simulink model "sistemaDesacopladoEquivalenteControlCorriente"  (R2012b)
settings: Solver=ode45  StartTime=0.0  StopTime=10.0  RelTol=1e-3
values from neighbouring files (symbols this model uses):
  b_m = bm+(bl/r^2)    (= 1.5e-05)    [InicializaYconstantes.m]
  J_m = Jm+(Jl/r^2)    (= 5.65099476805e-06)    [InicializaYconstantes.m]
  lambda = 0.01546    [InicializaYconstantes.m]
  Ld = 6.6*10^-3    (= 0.0066)    [InicializaYconstantes.m]
  Lq = 5.8*10^-3    (= 0.0058)    [InicializaYconstantes.m]
  Pp = 3    [InicializaYconstantes.m]
  R1 = -p1i*Lq    (= 29)    [InicializaYconstantes.m]
  R2 = -p1i*Ld    (= 33)    [InicializaYconstantes.m]
  T_l = Tl/r    (= 0.00499521477515)    [InicializaYconstantes.m]
settings Model: Creator=usuario  LastModifiedBy=usuario

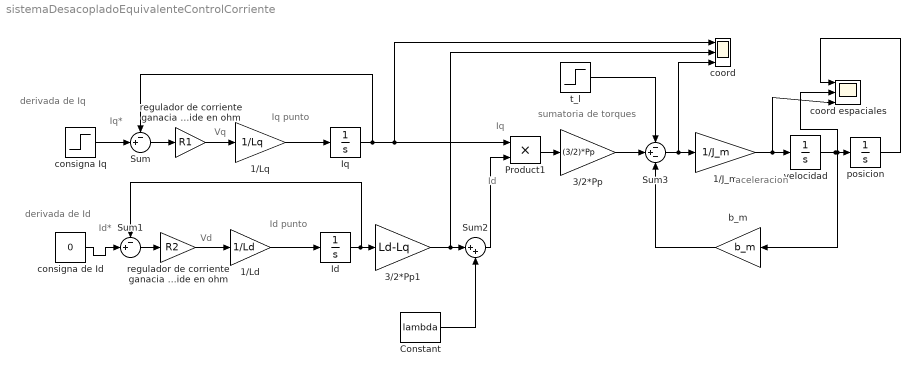
== system sistemaDesacopladoEquivalenteControlCorriente ==
  note: derivada de Id
  note: derivada de Iq
  note: Id*
  note: Iq*
  note: Vd
  note: Vq
  note: sumatoria de torques
  note: Iq
  note: aceleracion
  note: Id
  note: Iq punto
  note: Id punto
  1/J_m : Gain  Gain=1/J_m
  1/Ld : Gain  Gain=1/Ld
  1/Lq : Gain  Gain=1/Lq
  3/2*Pp : Gain  Gain=(3/2)*Pp
  3/2*Pp1 : Gain  Gain=Ld-Lq
  Constant : Constant  Value=lambda
  Id : Integrator
  Iq : Integrator
  Product1 : Product  RndMeth=Zero
  Sum : Sum  Inputs=-+|
  Sum1 : Sum  Inputs=-+|
  Sum2 : Sum  Inputs=|++
  Sum3 : Sum  Inputs=-+-
  b_m : Gain  Gain=b_m
  consigna Iq : Step  Time=0.1  After=.16  SampleTime=0
  consigna de Id : Constant  Value=0
  "coord " : Scope  NumInputPorts=3
      settings: TimeRange=10  YMin=0~-1~0  YMax=6~1~0.4  MaxDataPoints=8000
  coord espaciales : Scope  NumInputPorts=3
      settings: TimeRange=12  YMin=-1000~0~-50000  YMax=3000~300~100000  MaxDataPoints=8000
  posicion : Integrator
  regulador de corriente ganacia proporcional se mide en ohm : Gain  Gain=R2
  regulador de corriente ganacia proporcional1 se mide en ohm : Gain  Gain=R1
  t_l : Step  Time=.3  After=T_l  SampleTime=0
  velocidad : Integrator  ContinuousStateAttributes='velocidad'
  wires:
  3/2*Pp1/1 -> "coord "/2, Sum2/1
  Constant/1 -> Sum2/2
  Sum2/1 -> Product1/2
  Product1/1 -> 3/2*Pp/1
  Sum3/1 -> "coord "/3, 1/J_m/1
  b_m/1 -> Sum3/3
  t_l/1 -> Sum3/1
  3/2*Pp/1 -> Sum3/2
  1/J_m/1 -> velocidad/1, coord espaciales/3
  posicion/1 -> coord espaciales/1
  velocidad/1 -> coord espaciales/2, b_m/1, posicion/1
  regulador de corriente ganacia proporcional1 se mide en ohm/1 -> 1/Lq/1
  1/Lq/1 -> Iq/1
  Iq/1 -> Sum/1, Product1/1, "coord "/1
  Sum/1 -> regulador de corriente ganacia proporcional1 se mide en ohm/1
  consigna Iq/1 -> Sum/2
  Sum1/1 -> regulador de corriente ganacia proporcional se mide en ohm/1
  consigna de Id/1 -> Sum1/2
  1/Ld/1 -> Id/1
  regulador de corriente ganacia proporcional se mide en ohm/1 -> 1/Ld/1
  Id/1 -> Sum1/1, 3/2*Pp1/1
